simulink model "CanCRCcontorl3"  (R2018b)
settings: Solver=FixedStepDiscrete  StartTime=0.0  StopTime=2  FixedStep=0.01  RelTol=1e-3
PreLoadFcn:
  | librarySetup
  | eval([bdroot,'_startup']) %Calling [modelName]_startup.m
undefined symbols (not defined in the file or in its folder): byte_4, byte_5, byte_6, byte_7, CON4, D13, HANtuneOverride, LED1, Steer_Automation_Requested, Steer_Request, Steering_input, Throttle_input, Torque_Automation_Requested
libraries: HANcoder_STM32_Target x11, simulink x3, canmsglib x1
CloseFcn:
  | rtwprivate ssgencode ModelCloseRequest mytest
settings Model: Creator=Jason van Kolfschoten  LastModifiedBy=teus
settings SolverCC: PositivePriorityOrder=on
settings DataIOCC: LimitDataPoints=on  SaveFormat=Array  SignalLoggingSaveFormat=ModelDataLogs  SaveOutput=off  SaveTime=off
settings OptimizationCC: BlockReduction=off  DefaultParameterBehavior=Inlined  DefaultUnderspecifiedDataType=single  InlineInvariantSignals=on  ExpressionDepthLimit=2147483647  StateBitsets=on  DataBitsets=on  ZeroExternalMemoryAtStartup=off  ZeroInternalMemoryAtStartup=off  InitFltsAndDblsToZero=on  NoFixptDivByZeroProtection=on  EfficientFloat2IntCast=on  LifeSpan=inf
settings DebuggingCC: SaveWithDisabledLinksMsg=none  SaveWithParameterizedLinksMsg=none  CheckSSInitialOutputMsg=off  UnderspecifiedInitializationDetection=Classic  MergeDetectMultiDrivingBlocksExec=none  SignalResolutionControl=TryResolveAll  SolverPrmCheckMsg=warning  InheritedTsInSrcMsg=none  MultiTaskDSMMsg=warning  MultiTaskCondExecSysMsg=none  ParameterPrecisionLossMsg=none  FcnCallInpInsideContextMsg=warning  StateNameClashWarn=warning  SFUnexpectedBacktrackingDiag=warning  SFNoUnconditionalDefaultTransitionDiag=warning  SFExecutionAtInitializationDiag=none
settings HardwareCC: ProdBitPerPointer=32  ProdBitPerSizeT=32  ProdBitPerPtrDiffT=32  ProdLargestAtomicInteger=Long  ProdLargestAtomicFloat=Double  ProdWordSize=32  ProdHWDeviceType=ARM Compatible->ARM Cortex  TargetEndianess=LittleEndian  TargetHWDeviceType=Infineon->TriCore
settings ModelReferenceCC: PropagateSignalLabelsOutOfModel=off
settings SFSimCC: SimUseLocalCustomCode=off  MATLABDynamicMemAlloc=off
settings RTWCC: SystemTargetFile=ert.tlc  MakeCommand=make_rtw SHELL= HANcoder_PORTABLE=1 HANcoder_BOOTLOADER=1  TemplateMakefile=Olimexino_STM32_gcc.tmf  Description=Real-Time Workshop Embedded Coder (no auto configuration)  RTWUseLocalCustomCode=off
settings CodeAppCC: ForceParamTrailComments=on  IgnoreCustomStorageClasses=off  SimulinkDataObjDesc=on  CustomSymbolStrGlobalVar=rt$N$M  CustomSymbolStrType=$N$M  CustomSymbolStrFcn=$N$M$F  CustomSymbolStrMacro=$N$M  InsertBlockDesc=on  StateflowObjectComments=on  InternalIdentifier=Classic
settings ERTTargetCC: TargetFcnLib=ansi_tfl_tmw.mat  MultiwordLength=2048  IncludeMdlTerminateFcn=off  SuppressErrorStatus=on  SupportNonFinite=off  GenerateASAP2=on  InlinedParameterPlacement=NonHierarchical  ERTCustomFileTemplate=example_file_process.tlc  ConvertIfToSwitch=off  SuppressUnreachableDefaultCases=off
settings ConfigComp: CovMetricSettings=dw  CovHtmlReporting=on  CovSaveCumulativeToWorkspaceVar=on  CovSaveSingleToWorkspaceVar=on  CovExternalEMLEnable=off  CovSFcnEnable=off  DVMaxProcessTime=600  DVDisplayUnsatisfiableObjectives=on  DVAutomaticStubbing=off  DVSubSystemToStub=7.76600366011452e-316  DVParameterNames=7.76600366011452e-316  DVParameterConstraints=7.76600366011452e-316  DVParameterUseInAnalysis=7.76600366011452e-316  DVModelCoverageObjectives=MCDC  DVMaxTestCaseSteps=500  DVTestSuiteOptimization=CombinedObjectives  DVDetectActiveLogic=on  DVSaveHarnessModel=on

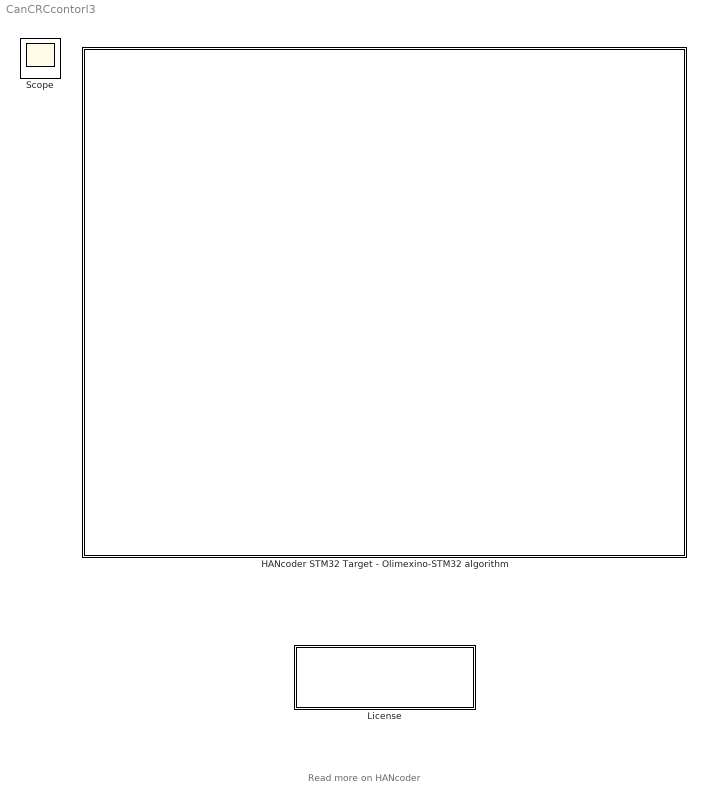
== system CanCRCcontorl3 ==
  note: Read more on HANcoder
  HANcoder STM32 Target - Olimexino-STM32 algorithm : Subsystem  mask(TopLevelSubsystem){}
      settings: CopyFcn=HANcoderChecks('Copy');  NameChangeFcn=HANcoderChecks('NameChangeOlimexino');  MoveFcn=HANcoderChecks('MoveOlimexino');
      mask Display: image(imread('Olimexino_STM32_HAN.jpg'))
  License : Subsystem  mask(License){}
      settings: NameChangeFcn=HANcoderChecks('NameChangeLicenseBlock');  OpenFcn=winopen('License.pdf')  MoveFcn=HANcoderChecks('MoveLicenseBlock');
      mask Display: disp(['End-User License Agreement\n','please read before use']);
  Scope : Scope

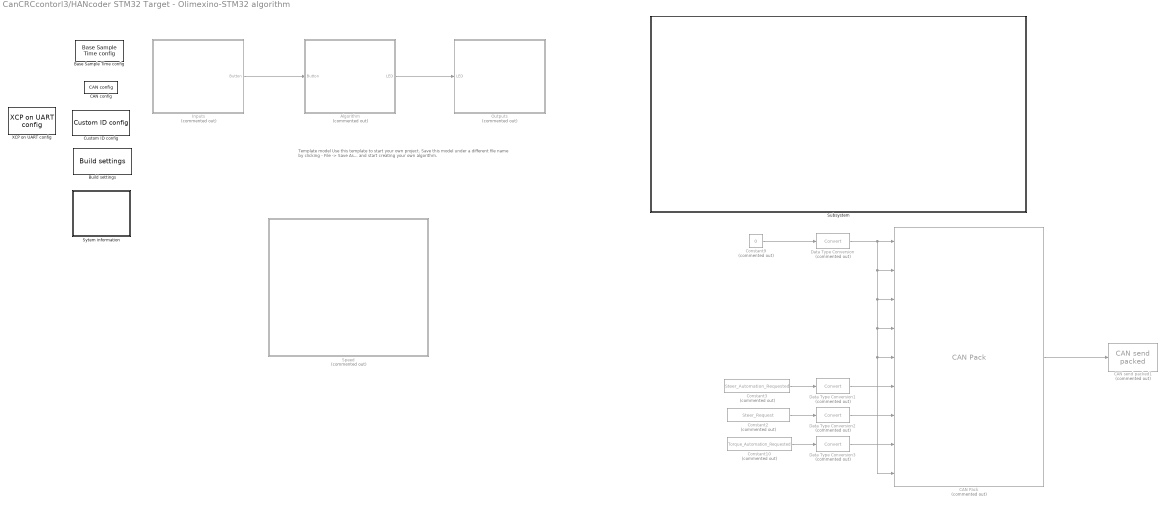
== system CanCRCcontorl3/HANcoder STM32 Target - Olimexino-STM32 algorithm ==
  note: Template model
      | Use this template to start your own project. Save this model
      | under a different file name by clicking - File -> Save As... and
      | start creating your own algorithm.
  Algorithm : Subsystem  Commented=on
  Base Sample Time config : HANcoder_STM32_Target/Olimexino STM32/System Config/Base Sample Time config  Tag=HANcoder_TARGET_STM32_Olimexino  Description=HANcoder Target STM32-Olimexino blockset version 1.1  baseSampleTime=10  extraStack=25
      settings: SourceProductName=HANcoder STM32 Target
  Build settings : HANcoder_STM32_Target/Olimexino STM32/System Config/Build settings  Tag=HANcoder_TARGET_STM32_Olimexino  AutoASAP2add=on  AutoFlash=CAN
      settings: SourceProductName=HANcoder STM32 Target
  CAN Pack : canmsglib/CAN Pack  Commented=on  CANdbFile=C:\Users\teus\Documents\twizzzy\peak usb\CAN file\Customer_Control_Diagnostics.dbc  MsgList=Customer_Control_1  MsgName=Customer_Control_1  MsgIDType=Standard (11-bit identifier)  MsgIdentifier=257  MsgLength=8  SignalInfo=Customer_Control_1_Alive$8$8$2$2$1$0$1$0$0$255$#Customer_Control_1_CRC$0$8$2$2$1$0$1$0$0$255$#Reserved_Byte_1$32$8$2$2$1$0$1$0$0$255$#Reserved_Byte_2$40$8$2$2$1$0$1$0$0$255$#Reserved_Byte_3$48$8$2$2$1$0$1$0$0$255$#Steer_Automation_Requested$56$1$2$2$1$0$1$0$0$1$#Steer_Request$16$8$2$1$1$0$1$0$-100$100$#Torque_Automation_Requested$60$1$2$2$1$0$1$0$0$1$#Torque_Request$24$8$2$1$1$0$1$0$-100$100$#  NSignals=9  StartBits=str2num('[int32(8);int32(0);int32(32);int32(40);int32(48);int32(56);int32(16);int32(60);int32(24)]')  SignalSizes=str2num('[int32(8);int32(8);int32(8);int32(8);int32(8);int32(1);int32(8);int32(1);int32(8)]')  ByteOrders=str2num('[int32(2);int32(2);int32(2);int32(2);int32(2);int32(2);int32(2);int32(2);int32(2)]')  DataTypes=str2num('[int32(2);int32(2);int32(2);int32(2);int32(2);int32(2);int32(1);int32(2);int32(1)]')  MultiplexTypes=str2num('[int32(1);int32(1);int32(1);int32(1);int32(1);int32(1);int32(1);int32(1);int32(1)]')  MultiplexValues=str2num('[double(0);double(0);double(0);double(0);double(0);double(0);double(0);double(0);double(0)]')  Factors=str2num('[double(1);double(1);double(1);double(1);double(1);double(1);double(1);double(1);double(1)]')  Offsets=str2num('[double(0);double(0);double(0);double(0);double(0);double(0);double(0);double(0);double(0)]')  Minimums=str2num('[double(0);double(0);double(0);double(0);double(0);double(0);double(-100);double(0);double(-100)]')  Maximums=str2num('[double(255);double(255);double(255);double(255);double(255);double(1);double(100);double(1);double(100)]')  Remote=off  ApplyMinMax=off  BusOutput=off
      settings: SourceProductName=Simulink Real-Time  SourceProductBaseCode=XP  DataFormat=CANdb specified signals
  CAN config : HANcoder_STM32_Target/Olimexino STM32/System Config/CAN config  Tag=HANcoder_TARGET_STM32_Olimexino  canBus1=on  baudRate1=500  rxMask1=hex2dec('00000000')  rxCode1=hex2dec('00000000')  rxMode1=Receive only 11-bit message identifiers  txBufSize1=32  evBufSize1=8
      settings: SourceProductName=HANcoder STM32 Target
  CAN send packed1 : HANcoder_STM32_Target/Olimexino STM32/CAN/CAN/CAN send packed  Tag=HANcoder_TARGET_STM32_Olimexino  Commented=on  canBus=CAN 1  tsamp=-1
      settings: SourceProductName=HANcoder STM32 Target
  Constant10 : Constant  Commented=on  Value=Torque_Automation_Requested  OutDataTypeStr=single  SampleTime=-1
  Constant2 : Constant  Commented=on  Value=Steer_Request  OutDataTypeStr=single  SampleTime=-1
  Constant3 : Constant  Commented=on  Value=Steer_Automation_Requested  OutDataTypeStr=single  SampleTime=-1
  Constant9 : Constant  Commented=on  Value=0  OutDataTypeStr=single  SampleTime=-1
  Custom ID config : HANcoder_STM32_Target/Olimexino STM32/System Config/Custom ID config  Tag=HANcoder_TARGET_STM32_Olimexino  softID=softwareID  softNUM=1
      settings: SourceProductName=HANcoder STM32 Target
  Data Type Conversion{,1..3} (4 alike) : DataTypeConversion  Commented=on
  Inputs : Subsystem  Commented=on
  Outputs : Subsystem  Commented=on
  Speed : Subsystem  Commented=on
  Subsystem : Subsystem
  Sytem information : Subsystem
  XCP on UART config : HANcoder_STM32_Target/Olimexino STM32/System Config/XCP on UART config  Tag=HANcoder_TARGET_STM32_Olimexino  channel=UART2: D1 & D0  baudrate=115200
      settings: SourceProductName=HANcoder STM32 Target
  wires:
  Inputs/1(Button) -> Algorithm/1(Button)
  Algorithm/1(LED) -> Outputs/1(LED)
  CAN Pack/1 -> CAN send packed1/1
  Data Type Conversion3/1 -> CAN Pack/8
  Data Type Conversion/1 -> CAN Pack/3, CAN Pack/4, CAN Pack/9, CAN Pack/5, CAN Pack/2, CAN Pack/1
  Constant3/1 -> Data Type Conversion1/1
  Constant2/1 -> Data Type Conversion2/1
  Constant9/1 -> Data Type Conversion/1
  Constant10/1 -> Data Type Conversion3/1
  Data Type Conversion1/1 -> CAN Pack/6
  Data Type Conversion2/1 -> CAN Pack/7

== system CanCRCcontorl3/License ==

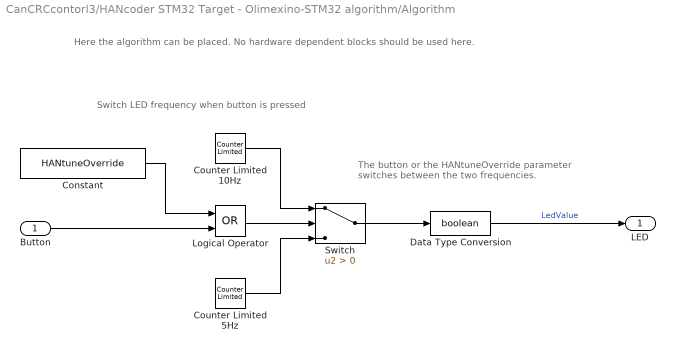
== system CanCRCcontorl3/HANcoder STM32 Target - Olimexino-STM32 algorithm/Algorithm ==
  note: The button or the HANtuneOverride parameter
      | switches between the two frequencies.
  note: Switch LED frequency when button is pressed
  note: Here the algorithm can be placed. No hardware dependent blocks should be used here.
  Button : Inport
  Constant : Constant  Value=HANtuneOverride  OutDataTypeStr=boolean
  Counter Limited 10Hz : simulink/Sources/Counter Limited  uplimit=1  tsamp=0.1
  Counter Limited 5Hz : simulink/Sources/Counter Limited  uplimit=1  tsamp=0.2
  Data Type Conversion : DataTypeConversion  OutDataTypeStr=boolean
  Logical Operator : Logic  Operator=OR  AllPortsSameDT=off  OutDataTypeStr=boolean
  Switch : Switch  Criteria=u2 > Threshold
  LED : Outport
  wires:
  Data Type Conversion/1 -> LED/1  "LedValue"
  Counter Limited 5Hz/1 -> Switch/3
  Switch/1 -> Data Type Conversion/1
  Button/1 -> Logical Operator/2
  Logical Operator/1 -> Switch/2
  Constant/1 -> Logical Operator/1
  Counter Limited 10Hz/1 -> Switch/1

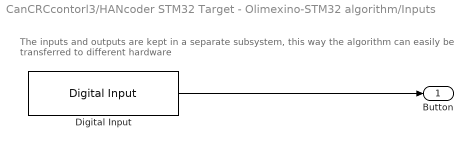
== system CanCRCcontorl3/HANcoder STM32 Target - Olimexino-STM32 algorithm/Inputs ==
  note: The inputs and outputs are kept in a separate subsystem, this way the algorithm can easily be transferred to different hardware
  Digital Input : HANcoder_STM32_Target/Olimexino STM32/Digital Inputs/Digital Input  Tag=HANcoder_TARGET_STM32_Olimexino  pinID=Pushbutton - BUT/BOOT0 - 5V Tolerant  config=Pulldown  tsamp=-1
      settings: SourceProductName=HANcoder STM32 Target
  Button : Outport
  wires:
  Digital Input/1 -> Button/1

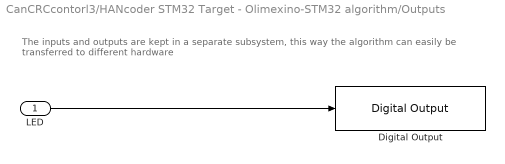
== system CanCRCcontorl3/HANcoder STM32 Target - Olimexino-STM32 algorithm/Outputs ==
  note: The inputs and outputs are kept in a separate subsystem, this way the algorithm can easily be transferred to different hardware
  LED : Inport
  Digital Output : HANcoder_STM32_Target/Olimexino STM32/Digital Outputs/Digital Output  Tag=HANcoder_TARGET_STM32_Olimexino  pinID=CON4 - D13/LED1  config=Push pull  tsamp=-1
      settings: SourceProductName=HANcoder STM32 Target
  wires:
  LED/1 -> Digital Output/1

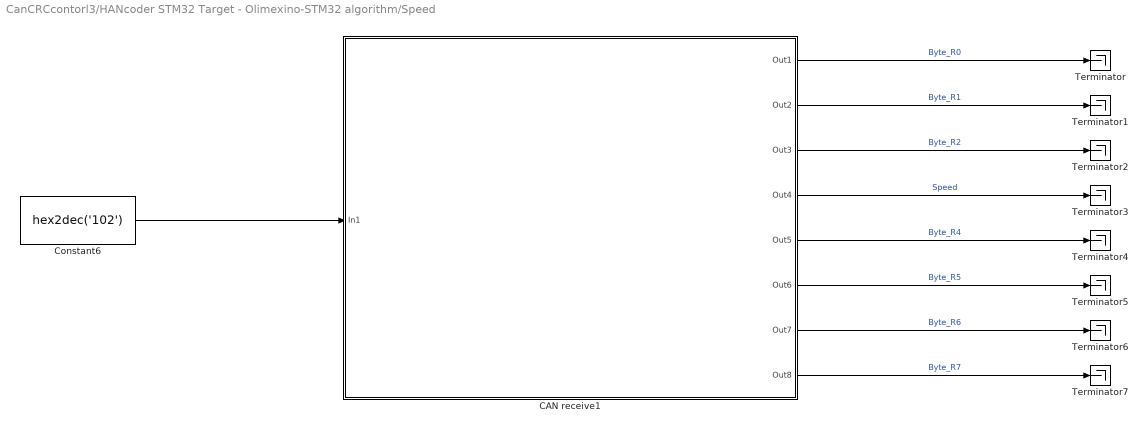
== system CanCRCcontorl3/HANcoder STM32 Target - Olimexino-STM32 algorithm/Speed ==
  CAN receive1 : Subsystem  Tag=HANcoder_TARGET_STM32_Olimexino  AncestorBlock=HANcoder_STM32_Target/Olimexino STM32/CAN/CAN/CAN receive  mask(CAN receive){canBus=CAN 1, outputNumber=7, dataType=uint8, byteOrder=off, tsamp=-1}
      mask prompts: canBus "CAN channel"; outputNumber "Output ports"; dataType "Output datatype"; byteOrder "Byte order: Checked = MSB first, unchecked = LSB first."; tsamp "Sample time"
      mask help:
      | Function
      | ==========
      | Receive the newest message from the specified CAN channel.
      |
      | Parameters
      | ==========
      | CAN channel:             The CAN channel to send the message on.
      | Output ports:             The amount of output ports
      | Output datatype:       The datatype of the output ports
      | Byte order:                 Select MSB or LSB first
      | Sample time:              -1 or divisible by base sample time [seconds]
      |
      | Input
      | ==========
      | Port 1:                       CAN ID(uint32) in hexadecimal ie: hex2dec('0a'),
      | to receive extended identifiers set the 32nd bit high (OR with 0x80000000)
      |
      | Output
      | ==========
      | Port 1:                       Checks for new message(int8)
      | Port 2..9                     Message data
      mask init:
      | sfcn_can_receive_mcb(canBus, outputNumber, dataType, byteOrder)
      settings: MoveFcn=drawLogos
      mask Help: web('sfcn_can_receive.html');
      mask TypeOptions canBus: CAN 1
      mask TypeOptions dataType: int8 | uint8 | int16 | uint16 | int32 | uint32 | boolean
      mask Display:
      | fprintf('Receive on\nCAN %x', canBus);
      | port_label('output', 1, 'new')
      | port_label('input', 1, 'ID');patch([435 441 441],[8 14 2],[1 0 0]);patch([443 443 449],[14 2 8],[0 0 0.35]);
  Constant6 : Constant  Value=hex2dec('102')  OutDataTypeStr=uint32  SampleTime=-1
  Terminator{,1..7} (8 alike) : Terminator
  wires:
  Constant6/1 -> CAN receive1/1(In1)
  CAN receive1/3(Out3) -> Terminator2/1  "Byte_R2"
  CAN receive1/4(Out4) -> Terminator3/1  "Speed"
  CAN receive1/2(Out2) -> Terminator1/1  "Byte_R1"
  CAN receive1/6(Out6) -> Terminator5/1  "Byte_R5"
  CAN receive1/1(Out1) -> Terminator/1  "Byte_R0"
  CAN receive1/5(Out5) -> Terminator4/1  "Byte_R4"
  CAN receive1/7(Out7) -> Terminator6/1  "Byte_R6"
  CAN receive1/8(Out8) -> Terminator7/1  "Byte_R7"

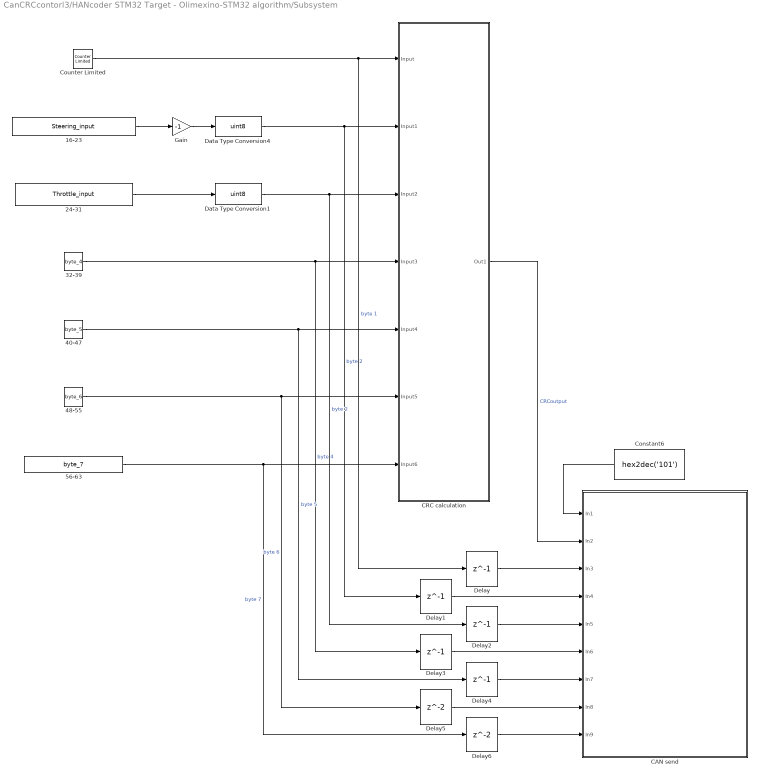
== system CanCRCcontorl3/HANcoder STM32 Target - Olimexino-STM32 algorithm/Subsystem ==
  16-23 : Constant  Value=Steering_input  OutDataTypeStr=int8  SampleTime=-1
  24-31 : Constant  Value=Throttle_input  OutDataTypeStr=int8  SampleTime=-1
  32-39 : Constant  Value=byte_4  OutDataTypeStr=uint8
  40-47 : Constant  Value=byte_5  OutDataTypeStr=uint8
  48-55 : Constant  Value=byte_6  OutDataTypeStr=uint8
  56-63 : Constant  Value=byte_7  OutDataTypeStr=uint8
  CAN send : Subsystem  Tag=HANcoder_TARGET_STM32_Olimexino  Priority=2  AncestorBlock=HANcoder_STM32_Target/Olimexino STM32/CAN/CAN/CAN send  mask(CAN send){canBus=CAN 1, frameType=Standard (11 bit), inputNumber=8, dataType=uint8, byteOrder=on, tsamp=-1}
      mask prompts: canBus "CAN channel"; frameType "Identifier type"; inputNumber "Input ports"; dataType "Input datatype"; byteOrder "Byte order: Checked = MSB first, unchecked = LSB first."; tsamp "Sample time"
      mask help:
      | Function
      | ==========
      | Send a message on the CAN channel.
      |
      | Parameters
      | ==========
      | CAN channel:           The CAN channel to send the message on.
      | Identifier type:         normal or extended ID's
      | Input ports:              The amount of input ports
      | Input datatype:        The datatype of the input ports
      | Byte order:               Select MSB or LSB first
      | Sample time:            -1 or divisible by base sample time [seconds]
      |
      | Input
      | ==========
      | Port 1:                   CAN ID(uint32) in hexadecimal ie: hex2dec('0a')
      | Port 2..9                CAN message data
      mask init:
      | sfcn_can_send_mcb(canBus, frameType, inputNumber, dataType, byteOrder)
      settings: MoveFcn=drawLogos
      mask Help: web('sfcn_can_send.html');
      mask TypeOptions canBus: CAN 1
      mask TypeOptions frameType: Standard (11 bit) | Extended (29 bit)
      mask TypeOptions dataType: int8 | uint8 | int16 | uint16 | int32 | uint32 | boolean
      mask Display:
      | fprintf('Send on\nCAN %x', canBus);
      | port_label('input', 1, 'ID');patch([250 256 256],[8 14 2],[1 0 0]);patch([258 258 264],[14 2 8],[0 0 0.35]);
  CRC calculation : Subsystem
  Constant6 : Constant  Value=hex2dec('101')  OutDataTypeStr=uint32  SampleTime=-1
  Counter Limited : simulink/Sources/Counter Limited  uplimit=255  tsamp=-1
  Data Type Conversion1 : DataTypeConversion  OutDataTypeStr=uint8  ConvertRealWorld=Stored Integer (SI)
  Data Type Conversion4 : DataTypeConversion  OutDataTypeStr=uint8  ConvertRealWorld=Stored Integer (SI)
  Delay{,1..4} (5 alike) : Delay  DelayLength=1
  Delay5 : Delay  SampleTime=0.01
  Delay6 : Delay  SampleTime=0.01
  Gain : Gain  Gain=-1  OutDataTypeStr=int8
  wires:
  CRC calculation/1(Out1) -> CAN send/2(In2)  "CRCoutput"
  Counter Limited/1 -> Delay/1, CRC calculation/1(Input)  "byte 1"
  24-31/1 -> Data Type Conversion1/1
  40-47/1 -> CRC calculation/5(Input4), Delay4/1  "byte 5"
  Data Type Conversion4/1 -> CRC calculation/2(Input1), Delay1/1  "byte 2"
  56-63/1 -> Delay6/1, CRC calculation/7(Input6)  "byte 7"
  32-39/1 -> CRC calculation/4(Input3), Delay3/1  "byte 4"
  16-23/1 -> Gain/1
  Constant6/1 -> CAN send/1(In1)
  48-55/1 -> CRC calculation/6(Input5), Delay5/1  "byte 6"
  Delay/1 -> CAN send/3(In3)
  Delay1/1 -> CAN send/4(In4)
  Delay2/1 -> CAN send/5(In5)
  Delay3/1 -> CAN send/6(In6)
  Delay4/1 -> CAN send/7(In7)
  Delay5/1 -> CAN send/8(In8)
  Delay6/1 -> CAN send/9(In9)
  Data Type Conversion1/1 -> CRC calculation/3(Input2), Delay2/1  "byte 2"
  Gain/1 -> Data Type Conversion4/1

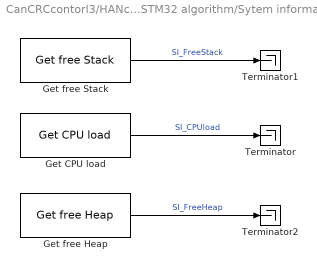
== system CanCRCcontorl3/HANcoder STM32 Target - Olimexino-STM32 algorithm/Sytem information ==
  Get CPU load : HANcoder_STM32_Target/Olimexino STM32/System Management/Get CPU load  Tag=HANcoder_TARGET_STM32_Olimexino  mode=Current CPU load  tsamp=-1
      settings: SourceProductName=HANcoder STM32 Target
  Get free Heap : HANcoder_STM32_Target/Olimexino STM32/System Management/Get free Heap  Tag=HANcoder_TARGET_STM32_Olimexino  tsamp=-1
      settings: SourceProductName=HANcoder STM32 Target
  Get free Stack : HANcoder_STM32_Target/Olimexino STM32/System Management/Get free Stack  Tag=HANcoder_TARGET_STM32_Olimexino  taskIdx=Application Control Task  tsamp=-1
      settings: SourceProductName=HANcoder STM32 Target
  Terminator : Terminator
  Terminator1 : Terminator
  Terminator2 : Terminator
  wires:
  Get CPU load/1 -> Terminator/1  "SI_CPUload"
  Get free Stack/1 -> Terminator1/1  "SI_FreeStack"
  Get free Heap/1 -> Terminator2/1  "SI_FreeHeap"

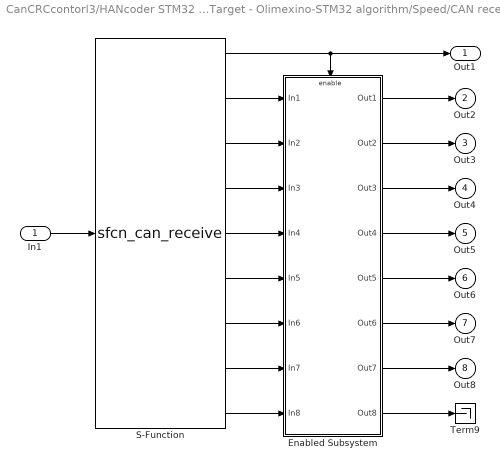
== system CanCRCcontorl3/HANcoder STM32 Target - Olimexino-STM32 algorithm/Speed/CAN receive1 ==
  In1 : Inport
  Enabled Subsystem : Subsystem  TreatAsAtomicUnit=on
  S-Function : M-S-Function  FunctionName=sfcn_can_receive  Parameters=tsamp, canBus, outputNumber, dataType, byteOrder
  Term9 : Terminator
  Out1 : Outport
  Out2 : Outport  Port=2
  Out3 : Outport  Port=3
  Out4 : Outport  Port=4
  Out5 : Outport  Port=5
  Out6 : Outport  Port=6
  Out7 : Outport  Port=7
  Out8 : Outport  Port=8
  wires:
  Enabled Subsystem/8(Out8) -> Term9/1
  Enabled Subsystem/7(Out7) -> Out8/1
  Enabled Subsystem/6(Out6) -> Out7/1
  Enabled Subsystem/5(Out5) -> Out6/1
  Enabled Subsystem/4(Out4) -> Out5/1
  Enabled Subsystem/3(Out3) -> Out4/1
  Enabled Subsystem/2(Out2) -> Out3/1
  Enabled Subsystem/1(Out1) -> Out2/1
  S-Function/7 -> Enabled Subsystem/6(In6)
  S-Function/8 -> Enabled Subsystem/7(In7)
  S-Function/4 -> Enabled Subsystem/3(In3)
  S-Function/3 -> Enabled Subsystem/2(In2)
  S-Function/2 -> Enabled Subsystem/1(In1)
  S-Function/9 -> Enabled Subsystem/8(In8)
  S-Function/5 -> Enabled Subsystem/4(In4)
  S-Function/6 -> Enabled Subsystem/5(In5)
  S-Function/1 -> Out1/1, Enabled Subsystem/Enable
  In1/1 -> S-Function/1

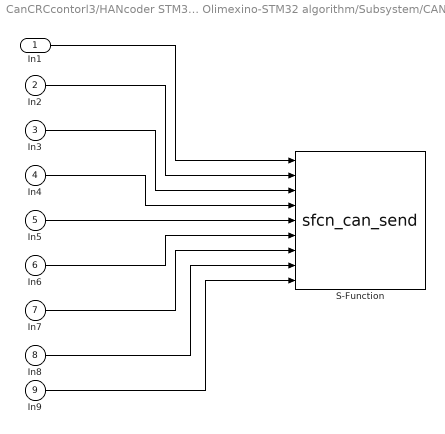
== system CanCRCcontorl3/HANcoder STM32 Target - Olimexino-STM32 algorithm/Subsystem/CAN send ==
  In1 : Inport
  In2 : Inport  Port=2
  In3 : Inport  Port=3
  In4 : Inport  Port=4
  In5 : Inport  Port=5
  In6 : Inport  Port=6
  In7 : Inport  Port=7
  In8 : Inport  Port=8
  In9 : Inport  Port=9
  S-Function : M-S-Function  FunctionName=sfcn_can_send  Parameters=tsamp, canBus, frameType, inputNumber, dataType, byteOrder
  wires:
  In9/1 -> S-Function/9
  In8/1 -> S-Function/8
  In7/1 -> S-Function/7
  In6/1 -> S-Function/6
  In5/1 -> S-Function/5
  In4/1 -> S-Function/4
  In3/1 -> S-Function/3
  In2/1 -> S-Function/2
  In1/1 -> S-Function/1

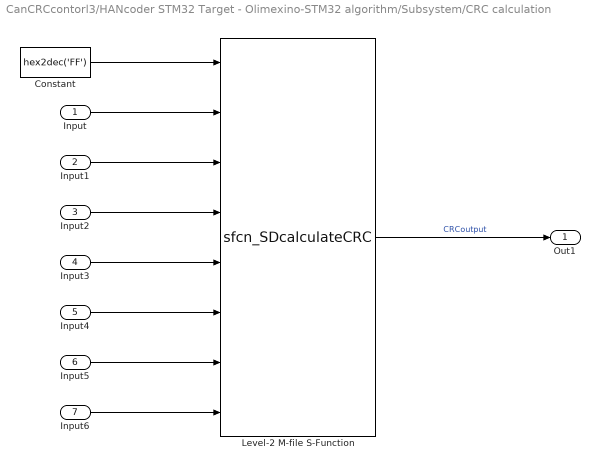
== system CanCRCcontorl3/HANcoder STM32 Target - Olimexino-STM32 algorithm/Subsystem/CRC calculation ==
  Input : Inport
  Input1 : Inport  Port=2
  Input2 : Inport  Port=3
  Input3 : Inport  Port=4
  Input4 : Inport  Port=5
  Input5 : Inport  Port=6
  Input6 : Inport  Port=7
  Constant : Constant  Value=hex2dec('FF')  OutDataTypeStr=uint8
  Level-2 M-file S-Function : M-S-Function  Priority=1  FunctionName=sfcn_SDcalculateCRC
  Out1 : Outport
  wires:
  Input5/1 -> Level-2 M-file S-Function/7
  Level-2 M-file S-Function/1 -> Out1/1  "CRCoutput"
  Input2/1 -> Level-2 M-file S-Function/4
  Constant/1 -> Level-2 M-file S-Function/1
  Input6/1 -> Level-2 M-file S-Function/8
  Input1/1 -> Level-2 M-file S-Function/3
  Input4/1 -> Level-2 M-file S-Function/6
  Input/1 -> Level-2 M-file S-Function/2
  Input3/1 -> Level-2 M-file S-Function/5

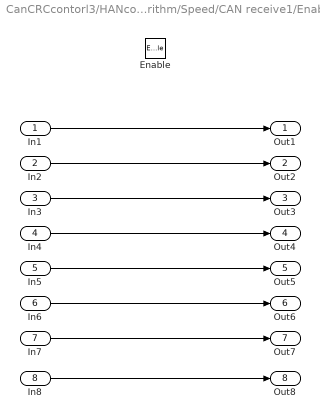
== system CanCRCcontorl3/HANcoder STM32 Target - Olimexino-STM32 algorithm/Speed/CAN receive1/Enabled Subsystem ==
  In1 : Inport
  In2 : Inport  Port=2
  In3 : Inport  Port=3
  In4 : Inport  Port=4
  In5 : Inport  Port=5
  In6 : Inport  Port=6
  In7 : Inport  Port=7
  In8 : Inport  Port=8
  Enable : EnablePort
  Out1 : Outport
  Out2 : Outport  Port=2
  Out3 : Outport  Port=3
  Out4 : Outport  Port=4
  Out5 : Outport  Port=5
  Out6 : Outport  Port=6
  Out7 : Outport  Port=7
  Out8 : Outport  Port=8
  wires:
  In8/1 -> Out8/1
  In7/1 -> Out7/1
  In6/1 -> Out6/1
  In5/1 -> Out5/1
  In4/1 -> Out4/1
  In3/1 -> Out3/1
  In2/1 -> Out2/1
  In1/1 -> Out1/1
